simulink model "trackHu"  (Simulink 6.3)
settings: Solver=ode45  StartTime=0.0  StopTime=1000  RelTol=1e-3
libraries: simulink x9
settings Model: LastModifiedBy=Administrator

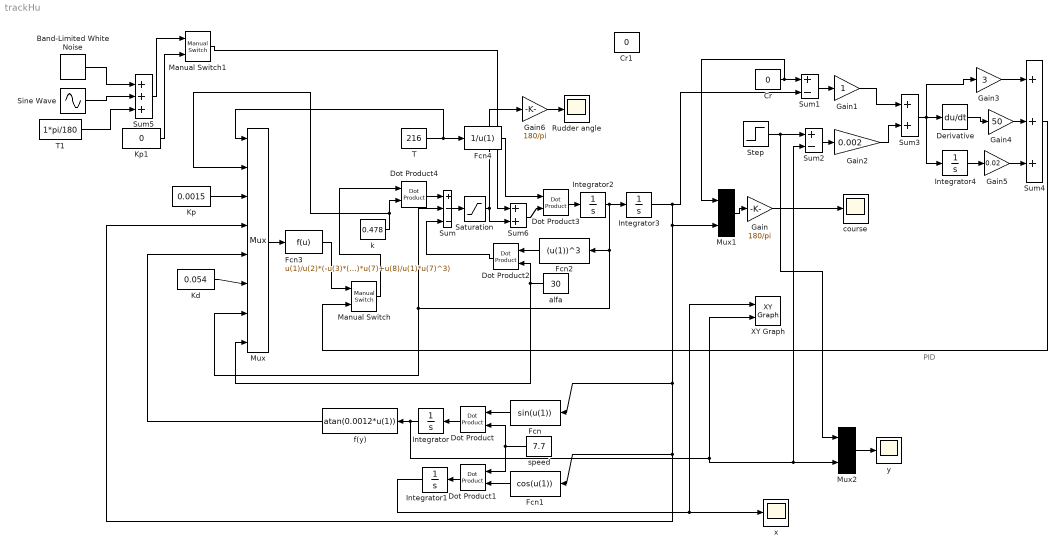
== system trackHu ==
  note: PID
  Band-Limited White Noise : simulink/Sources/Band-Limited White Noise  Cov=[0.1*pi/180]  Ts=0.1  seed=[23341]
  Cr : Constant  Value=0
  Cr1 : Constant  Value=0
  Derivative : Derivative
  Dot Product : simulink/Math Operations/Dot Product  Orientation=left  InputSameDT=on  OutDataType=sfix(16)  OutScaling=2^-10  DoSatur=off
  Dot Product1 : simulink/Math Operations/Dot Product  Orientation=left  InputSameDT=on  OutDataType=sfix(16)  OutScaling=2^-10  DoSatur=off
  Dot Product2 : simulink/Math Operations/Dot Product  Orientation=left  InputSameDT=on  OutDataType=sfix(16)  OutScaling=2^-10  DoSatur=off
  Dot Product3 : simulink/Math Operations/Dot Product  InputSameDT=on  OutDataType=sfix(16)  OutScaling=2^-10  DoSatur=off
  Dot Product4 : simulink/Math Operations/Dot Product  InputSameDT=on  OutDataType=sfix(16)  OutScaling=2^-10  DoSatur=off
  Fcn : Fcn  Orientation=left  Expr=sin(u(1))
  Fcn1 : Fcn  Orientation=left  Expr=cos(u(1))
  Fcn2 : Fcn  Orientation=left  Expr=(u(1))^3
  Fcn3 : Fcn  Expr=u(1)/u(2)*(-u(3)*(u(4)+u(5))-(u(6)-1/u(1))*u(7)+u(8)/u(1)*u(7)^3)
  Fcn4 : Fcn  Expr=1/u(1)
  Gain : Gain  Gain=180/pi
  Gain1 : Gain
  Gain2 : Gain  Gain=0.002
  Gain3 : Gain  Gain=3
  Gain4 : Gain  Gain=50
  Gain5 : Gain  Gain=0.02
  Gain6 : Gain  Gain=180/pi
  Integrator : Integrator  Orientation=left  InitialCondition=-1000
  Integrator1 : Integrator  Orientation=left
  Integrator2 : Integrator
  Integrator3 : Integrator  InitialCondition=160*pi/180
  Integrator4 : Integrator
  Kd : Constant  Value=0.054
  Kp : Constant  Value=0.0015
  Kp1 : Constant  Value=0
  Manual Switch : simulink/Signal Routing/Manual Switch  sw=1  action=0
  Manual Switch1 : simulink/Signal Routing/Manual Switch  sw=0  action=0
  Mux : Mux  Inputs=8
  Mux1 : Mux  Inputs=2
  Mux2 : Mux  Inputs=2
  Rudder angle : Scope
      settings: SaveName=ScopeData3
  Saturation : Saturate  UpperLimit=35*pi/180  LowerLimit=-35*pi/180
  Sine Wave : Sin  Amplitude=0.0  Frequency=2*pi/400  SampleTime=0
  Step : Step  Time=0  After=0  SampleTime=0
  Sum : Sum  Inputs=+--
  Sum1 : Sum  Inputs=+-
  Sum2 : Sum  Inputs=+-
  Sum3 : Sum
  Sum4 : Sum  Inputs=+++
  Sum5 : Sum  Inputs=+++
  Sum6 : Sum
  T : Constant  Value=216
  T1 : Constant  Value=1*pi/180
  XY Graph : simulink/Sinks/XY Graph  xmin=-500  xmax=6000  ymin=-1000  ymax=200  st=-1
  alfa : Constant  Orientation=left  Value=30
  course : Scope
      settings: YMin=-70  YMax=0
  f(y) : Fcn  Orientation=left  Expr=atan(0.0012*u(1))
  k : Constant  Value=0.478
  speed : Constant  Orientation=left  Value=7.7
  x : Scope
  y : Scope
      settings: YMin=-1750  YMax=500  SaveName=ScopeData2
  wires:
  Fcn/1 -> Dot Product/1
  speed/1 -> Dot Product/2, Dot Product1/1
  Fcn1/1 -> Dot Product1/2
  Dot Product/1 -> Integrator/1
  Dot Product1/1 -> Integrator1/1
  Integrator2/1 -> Integrator3/1, Fcn2/1, Sum/2, Mux/7
  Integrator3/1 -> Sum1/2, Fcn/1, Fcn1/1, Mux/4, Mux1/2
  Sum/1 -> Saturation/1
  Dot Product3/1 -> Integrator2/1
  Dot Product4/1 -> Sum/1
  Fcn2/1 -> Dot Product2/1
  alfa/1 -> Dot Product2/2, Mux/8
  Dot Product2/1 -> Sum/3
  Integrator/1 -> f(y)/1, XY Graph/2, Sum2/2, Mux2/2
  k/1 -> Dot Product4/2, Mux/2
  T/1 -> Fcn4/1, Mux/1
  Fcn4/1 -> Dot Product3/1
  Kp/1 -> Mux/3
  Kd/1 -> Mux/6
  f(y)/1 -> Mux/5
  Mux/1 -> Fcn3/1
  Gain/1 -> course/1
  Integrator1/1 -> x/1, XY Graph/1
  Cr/1 -> Sum1/1, Mux1/1
  Sum1/1 -> Gain1/1
  Step/1 -> Sum2/1, Mux2/1
  Sum2/1 -> Gain2/1
  Gain1/1 -> Sum3/1
  Gain2/1 -> Sum3/2
  Sum3/1 -> Derivative/1, Integrator4/1, Gain3/1
  Derivative/1 -> Gain4/1
  Integrator4/1 -> Gain5/1
  Gain3/1 -> Sum4/1
  Gain4/1 -> Sum4/2
  Gain5/1 -> Sum4/3
  Fcn3/1 -> Manual Switch/1
  Manual Switch/1 -> Dot Product4/1
  Sum4/1 -> Manual Switch/2
  Gain6/1 -> Rudder angle/1
  Saturation/1 -> Gain6/1, Sum6/2
  Mux1/1 -> Gain/1
  Mux2/1 -> y/1
  Band-Limited White Noise/1 -> Sum5/1
  Sine Wave/1 -> Sum5/2
  T1/1 -> Sum5/3
  Sum6/1 -> Dot Product3/2
  Sum5/1 -> Manual Switch1/1
  Kp1/1 -> Manual Switch1/2
  Manual Switch1/1 -> Sum6/1
